simulink model "model"  (R2015a)
settings: Solver=ode45  StartTime=0.0  StopTime=10.0  RelTol=1e-3
values from neighbouring files (symbols this model uses):
  b = Kf    (= 0.01)    [init.m]    (also in main.m)
  J = 0.02    [init.m]    (also in main.m)
  K = Kb    (= 0.1)    [init.m]    (also in main.m = place(A,B,[p1 p2]))
  Kb = 0.1    [init.m]    (also in main.m)
  Kf = 0.01    [init.m]    (also in main.m)
  Km = 0.1    [init.m]    (also in main.m)
  L = 0.5    [init.m]    (also in main.m)
  R = 2.0    (= 2)    [init.m]    (also in main.m)
libraries: fuzblock x1, commnoisgen2 x1
settings Model: Creator=dsp520  LastModifiedBy=dsp520

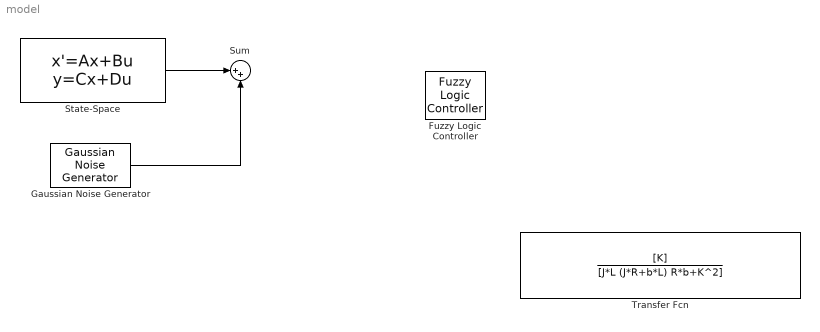
== system model ==
  Fuzzy Logic Controller : fuzblock/Fuzzy Logic  Controller  fis=[]
  Gaussian Noise Generator : commnoisgen2/Gaussian Noise Generator  m=0  d=1  s=41  Ts=1  frameBased=off  sampPerFrame=1  orient=off  outDataType=double
  State-Space : StateSpace  A=[-R/L -Kb/L; Km/J -Kf/J]  B=[1/L; 0]  C=[0 1]  D=[0]  X0=[0 0]
  Sum : Sum  Inputs=|++
  Transfer Fcn : TransferFcn  Numerator=[K]  Denominator=[J*L (J*R+b*L) R*b+K^2]
  wires:
  State-Space/1 -> Sum/1
  Gaussian Noise Generator/1 -> Sum/2
